simulink model "nonlineardtm"  (R2018b)
settings: configuration reference "Physics" (kept outside this file)
model workspace (MAT data in the model file):
  MCOS : class17 (value not decoded)
undefined symbols (not defined in the file): Aerodynamics, Aligning, Antisway, Brakes, Compliance, ContactPatch, Environment, k1_TireFB_PT1, k1_WheelsFB_PT1, k2_TireFB_PT1, Kinematics, Lateral, Longitudinal, normalizeAngle, omega0_K_Vehicle_radps, omega0_Wheels_radps, Overturning, p_Tires_Pa, Rolling, Scaling, SensorData, Structural, TireSimulation, Turnslip, v0_K_Vehicle_mps, v0z_Wheels_mps, VehicleData, Vertical, Wheels, x0_verticaldynamics, z0_TireDeflection_m
libraries: vehdynlibtire x4, vehdynlibsuspension x2, vrlib x1, vehdynlibeom x1
(part 3 of 5)

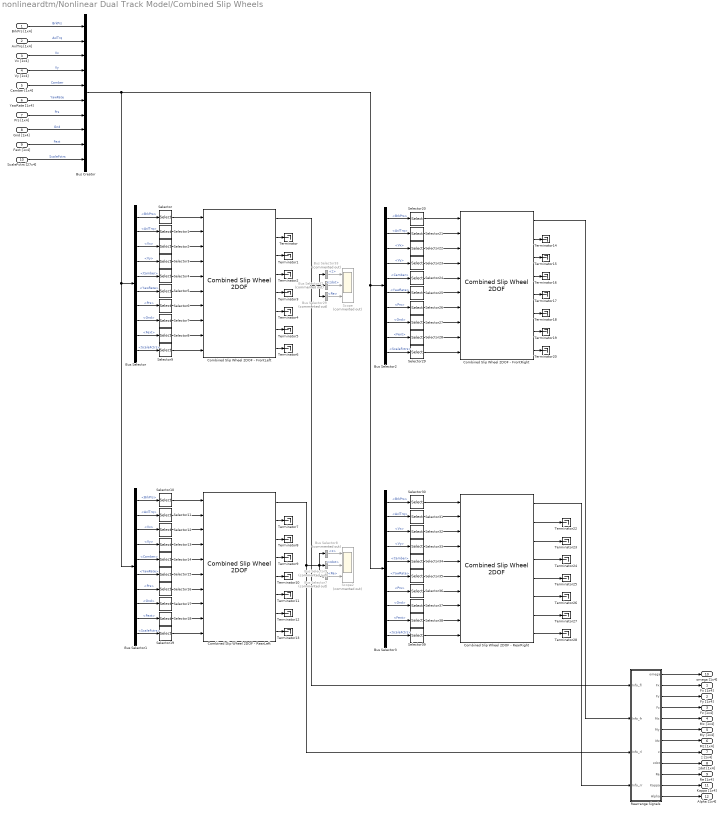
== system nonlineardtm/Nonlinear Dual Track Model/Combined Slip Wheels ==
  BrkPrs [1x4] : Inport
  AxlTrq [1x4] : Inport  Port=2
  Vx [1x4] : Inport  Port=3
  Vy [1x4] : Inport  Port=4
  Camber [1x4] : Inport  Port=5
  YawRate [1x4] : Inport  Port=6
  Prs [1x4] : Inport  Port=7
  Gnd [1x4] : Inport  Port=8
  Fext [1x4] : Inport  Port=9
  ScaleFctrs [27x4] : Inport  Port=10
  Bus Creator : BusCreator  Inputs=10
  Bus Selector{,1..3} (4 alike) : BusSelector  OutputSignals=BrkPrs,AxlTrq,Vx,Vy,Camber,YawRate,Prs,Gnd,Fext,ScaleFctrs
  Bus Selector29 : BusSelector  Commented=on  OutputSignals=Re
  Bus Selector33 : BusSelector  Commented=on  OutputSignals=z
  Bus Selector37 : BusSelector  Commented=on  OutputSignals=zdot
  Bus Selector7 : BusSelector  Commented=on  OutputSignals=Re
  Bus Selector8 : BusSelector  Commented=on  OutputSignals=z
  Bus Selector9 : BusSelector  Commented=on  OutputSignals=zdot
  Combined Slip Wheel 2DOF - FrontLeft : vehdynlibtire/Combined Slip Wheel 2DOF  BrakeType=Disc  mu_static=Brakes.mue_BrakePadsStaticFB (1)  mu_kinetic=Brakes.mue_BrakePadsKineticFB (1)  disk_abore=Brakes.d_BrakeBoreDiameterFB_m (1)  Rm=Brakes.r_BrakePadsMeanLeverRadiusFB_m (1)  num_pads=Brakes.n_BrakePadsNumberFB (1)  drum_abore=0.0508  drum_a=0.123  drum_c=0.212  drum_r=0.15  drum_theta1=0  drum_theta2=126  brake_p_bpt=[1 11.4736842105263 21.9473684210526 32.4210526315789 42.8947368421053 53.3684210526316 63.8421052631579 74.3157894736842 84.7894736842105 95.2631578947368 105.736842105263 116.210526315789 126.684210526316 137.157894736842 147.631578947368 158.105263157895 168.578947368421 179.052631578947 189.526315789474 200]  brake_n_bpt=[0 52.6315789473684 105.263157894737 157.894736842105 210.526315789474 263.157894736842 315.789473684211 368.421052631579 421.052631578947 473.684210526316 526.315789473684 578.947368421053 631.578947368421 684.210526315789 736.842105263158 789.473684210526 842.105263157895 894.736842105263 947.368421052632 1000]  f_brake_t=[43.4900602404453 42.5056030554862 41.5350898940194 40.5780454442085 39.6340111501808 38.7025443887544 37.7832176914519 36.8756180088306 35.9793460143796 35.0940154454303 34.2192524787115 33.3546951383474 32.4999927342521 31.6548053290159 30.8188032315107 29.991666515561 29.1730845621415 28.362755623661 27.5603864089927 26.765691687993;498.991217495636 487.695866636631 476.560505099801 465.579679307235 454.748127933653 444.060772460445 433.51270824929 423.099196101319 412.81565427025 402.657650900201 392.620896861006 382.701238955775 372.894653477208 363.197240090814 353.605216024701 344.114910546964 334.722759712992 325.425301366216 316.219170376863 307.10109410434;954.492374750826 932.886130217776 911.585920305583 890.581313170261 869.862244717126 849.419000532136 829.242198807128 809.322774193808 789.651962526121 770.221286354971 751.0225412433 732.047782773203 713.289314220164 694.739674852612 676.391628817892 658.238154578366 640.272434863842 622.48784710877 604.877954344734 587.436496520688;1409.99353200602 1378.07639379892 1346.61133551136 1315.58294703329 1284.9763615006 1254.77722860383 1224.97168936497 1195.5463522863 1166.48827078199 1137.78492180974 1109.42418562559 1081.39432659063 1053.68397496312 1026.28210961441 999.178041611083 972.361398609768 945.822110014692 919.550392851325 893.536738312604 867.771898937035;1865.49468926121 1823.26665738007 1781.63675071715 1740.58458089631 1700.09047828407 1660.13545667552 1620.7011799228 1581.76993037878 1543.32457903786 1505.34855726451 1467.82583000789 1430.74087040806 1394.07863570608 1357.82454437621 1321.96445440427 1286.48464264117 1251.37178516554 1216.61293859388 1182.19552228048 1148.10730135338;2320.9958465164 2268.45692096121 2216.66216592293 2165.58621475934 2115.20459506754 2065.49368474721 2016.43067048064 1967.99350847127 1920.16088729373 1872.91219271928 1826.22747439018 1780.08741422549 1734.47329644903 1689.36697913801 1644.75086719747 1600.60788667257 1556.92146031639 1513.67548433643 1470.85430624835 1428.44270376973;2776.49700377159 2713.64718454235 2651.68758112871 2590.58784862237 2530.31871185102 2470.8519128189 2412.16016103848 2354.21708656376 2296.9971955496 2240.47582817405 2184.62911877248 2129.43395804292 2074.86795719199 2020.9094138998 1967.53727999066 1914.73113070398 1862.47113546724 1810.73803007899 1759.51309021622 1708.77810618608;3231.99816102678 3158.8374481235 3086.71299633449 3015.58948248539 2945.43282863449 2876.21014089059 2807.88965159632 2740.44066465625 2673.83350380547 2608.03946362882 2543.03076315477 2478.78050186034 2415.26261793494 2352.4518486616 2290.32369278385 2228.85437473538 2168.02081061809 2107.80057582154 2048.17187418409 1989.11350860242;3687.49931828197 3604.02771170464 3521.73841154027 3440.59111634842 3360.54694541796 3281.56836896228 3203.61914215416 3126.66424274874 3050.66981206134 2975.60309908359 2901.43240753707 2828.12704567777 2755.6572786779 2683.9942834234 2613.11010557704 2542.97761876678 2473.57048576894 2404.8631215641 2336.83065815196 2269.44891101877;4143.00047553716 4049.21797528579 3956.76382674606 3865.59275021144 3775.66106220143 3686.92659703397 3599.34863271199 3512.88782084123 3427.50612031721 3343.16673453836 3259.83405191936 3177.4735894952 3096.05193942085 3015.5367181852 2935.89651837023 2857.10086279818 2779.12016091979 2701.92566730665 2625.48944211983 2549.78431343512;4598.50163279235 4494.40823886693 4391.78924195184 4290.59438407447 4190.77517898491 4092.28482510566 3995.07812326983 3899.11139893372 3804.34242857308 3710.73036999313 3618.23569630166 3526.82013331263 3436.44660016381 3347.079152947 3258.68293116342 3171.22410682959 3084.66983607064 2998.98821304921 2914.1482260877 2830.11971585147;5054.00279004754 4939.59850244808 4826.81465715762 4715.59601793749 4605.88929576838 4497.64305317735 4390.80761382767 4285.3349770262 4181.17873682896 4078.2940054479 3976.63734068395 3876.16667713006 3776.84126090677 3678.62158770879 3581.46934395661 3485.34735086099 ...(+2764 chars)]  tireParamSet=vdynPassCar.mat  plySteer=off  turnslip=off  PRESMAX=TireSimulation.PRESMAX(1)  PRESMIN=TireSimulation.PRESMIN(1)  FZMAX=TireSimulation.FZMAX(1)  FZMIN=TireSimulation.FZMIN(1)  VXLOW=TireSimulation.VXLOW(1)  KPUMAX=TireSimulation.KPUMAX(1)  KPUMIN=TireSimulation.KPUMIN(1)  ALPMAX=TireSimulation.ALPMAX(1)  ALPMIN=TireSimulation.ALPMIN(1)  CAMMAX=TireSimulation.CAMMAX(1)  CAMMIN=TireSimulation.CAMMIN(1)  LONGVL=TireSimulation.LONGVL(1)  omegao=omega0_Wheels_radps(1)  br=Wheels.mue_Wheels(1)  UNLOADED_RADIUS=Wheels.UNLOADED_RADIUS(1)  NOMPRES=Wheels.NOMPRES(1)  FNOMIN=Wheels.FNOMIN(1)  WIDTH=Wheels.WIDTH(1)  MASS=Wheels.m_WheelsFB_kg (1)  IYY=Wheels.Iyy_WheelsFB_kgm2 (1)  GRAVITY=- Wheels.a_Gravity_mps2  zo=z0_TireDeflection_m(1)  zdoto=v0z_Wheels_mps(1)  BREFF=Vertical.BREFF(1)  DREFF=Vertical.DREFF(1)  FREFF=Vertical.FREFF(1)  Q_RE0=Vertical.Q_RE0(1)  Q_V1=Vertical.Q_V1(1)  Q_V2=Vertical.Q_V2(1)  Q_FZ1=Vertical.Q_FZ1(1)  Q_FZ2=Vertical.Q_FZ2(1)  Q_FZ3=Vertical.Q_FZ3(1)  Q_FCX=Vertical.Q_FCX(1)  Q_FCY=Vertical.Q_FCY(1)  Q_FCY2=Vertical.Q_FCY2(1)  PFZ1=Vertical.PFZ1(1)  VERTICAL_STIFFNESS=Vertical.VERTICAL_STIFFNESS(1)  VERTICAL_DAMPING=Vertical.VERTICAL_DAMPING(1)  LONGITUDINAL_STIFFNESS=Structural.LONGITUDINAL_STIFFNESS(1)  LATERAL_STIFFNESS=Structural.LATERAL_STIFFNESS(1)  PCFX1=Structural.PCFX1(1)  PCFX2=Structural.PCFX2(1)  PCFX3=Structural.PCFX3(1)  PCFY1=Structural.PCFY1(1)  PCFY2=Structural.PCFY2(1)  PCFY3=Structural.PCFY3(1)  Q_RA1=ContactPatch.Q_RA1(1)  Q_RA2=ContactPatch.Q_RA2(1)  Q_RB1=ContactPatch.Q_RB1(1)  Q_RB2=ContactPatch.Q_RB2(1)  PCX1=Longitudinal.PCX1(1)  PDX1=Longitudinal.PDX1(1)  PDX2=Longitudinal.PDX2(1)  PDX3=Longitudinal.PDX3(1)  PEX1=Longitudinal.PEX1(1)  PEX2=Longitudinal.PEX2(1)  PEX3=Longitudinal.PEX3(1)  PEX4=Longitudinal.PEX4(1)  PKX1=Longitudinal.PKX1(1)  PKX2=Longitudinal.PKX2(1)  PKX3=Longitudinal.PKX3(1)  PHX1=Longitudinal.PHX1(1)  PHX2=Longitudinal.PHX2(1)  PVX1=Longitudinal.PVX1(1)  PVX2=Longitudinal.PVX2(1)  PPX1=Longitudinal.PPX1(1)  PPX2=Longitudinal.PPX2(1)  PPX3=Longitudinal.PPX3(1)  PPX4=Longitudinal.PPX4(1)  RBX1=Longitudinal.RBX1(1)  RBX2=Longitudinal.RBX2(1)  RBX3=Longitudinal.RBX3(1)  RCX1=Longitudinal.RCX1(1)  REX1=Longitudinal.REX1(1)  REX2=Longitudinal.REX2(1)  RHX1=Longitudinal.RHX1(1)  QSX1=Overturning.QSX1(1)  QSX2=Overturning.QSX2(1)  QSX3=Overturning.QSX3(1)  QSX4=Overturning.QSX4(1)  QSX5=Overturning.QSX5(1)  QSX6=Overturning.QSX6(1)  QSX7=Overturning.QSX7(1)  QSX8=Overturning.QSX8(1)  QSX9=Overturning.QSX9(1)  QSX10=Overturning.QSX10(1)  QSX11=Overturning.QSX11(1)  QSX12=Overturning.QSX12(1)  QSX13=Overturning.QSX13(1)  QSX14=Overturning.QSX14(1)  PPMX1=Overturning.PPMX1(1)  PCY1=Lateral.PCY1(1)  PDY1=Lateral.PDY1(1)  PDY2=Lateral.PDY2(1)  PDY3=Lateral.PDY3(1)  PEY1=Lateral.PEY1(1)  PEY2=Lateral.PEY2(1)  PEY3=Lateral.PEY3(1)  PEY4=Lateral.PEY4(1)  PEY5=Lateral.PEY5(1)  PKY1=Lateral.PKY1(1)  PKY2=Lateral.PKY2(1)  PKY3=Lateral.PKY3(1)  PKY4=Lateral.PKY4(1)  PKY5=Lateral.PKY5(1)  PKY6=Lateral.PKY6(1)  PKY7=Lateral.PKY7(1)  PHY1=Lateral.PHY1(1)  PHY2=Lateral.PHY2(1)  PVY1=Lateral.PVY1(1)  PVY2=Lateral.PVY2(1)  PVY3=Lateral.PVY3(1)  PVY4=Lateral.PVY4(1)  PPY1=Lateral.PPY1(1)  PPY2=Lateral.PPY2(1)  PPY3=Lateral.PPY3(1)  PPY4=Lateral.PPY4(1)  PPY5=Lateral.PPY5(1)  RBY1=Lateral.RBY1(1)  RBY2=Lateral.RBY2(1)  RBY3=Lateral.RBY3(1)  RBY4=Lateral.RBY4(1)  RCY1=Lateral.RCY1(1)  REY1=Lateral.REY1(1)  REY2=Lateral.REY2(1)  RHY1=Lateral.RHY1(1)  RHY2=Lateral.RHY2(1)  RVY1=Lateral.RVY1(1)  RVY2=Lateral.RVY2(1)  RVY3=Lateral.RVY3(1)  RVY4=Lateral.RVY4(1)  RVY5=Lateral.RVY5(1)  RVY6=Lateral.RVY6(1)  QSY1=Rolling.QSY1(1)  QSY2=Rolling.QSY2(1)  QSY3=Rolling.QSY3(1)  QSY4=Rolling.QSY4(1)  QSY5=Rolling.QSY5(1)  QSY6=Rolling.QSY6(1)  QSY7=Rolling.QSY7(1)  QSY8=Rolling.QSY8(1)  QBZ1=Aligning.QBZ1(1)  QBZ2=Aligning.QBZ2(1)  QBZ3=Aligning.QBZ3(1)  QBZ4=Aligning.QBZ4(1)  QBZ5=Aligning.QBZ5(1)  QBZ6=Aligning.QBZ6(1)  QBZ9=Aligning.QBZ9(1)  QBZ10=Aligning.QBZ10(1)  QCZ1=Aligning.QCZ1(1)  QDZ1=Aligning.QDZ1(1)  QDZ2=Aligning.QDZ2(1)  QDZ3=Aligning.QDZ3(1)  QDZ4=Aligning.QDZ4(1)  QDZ6=Aligning.QDZ6(1)  QDZ7=Aligning.QDZ7(1)  QDZ8=Aligning.QDZ8(1)  QDZ9=Aligning.QDZ9(1)  QDZ10=Aligning.QDZ10(1)  QDZ11=Aligning.QDZ11(1)  QEZ1=Aligning.QEZ1(1)  QEZ2=Aligning.QEZ2(1)  QEZ3=Aligning.QEZ3(1)  QEZ4=Aligning.QEZ4(1)  QEZ5=Aligning.QEZ5(1)  QHZ1=Aligning.QHZ1(1)  QHZ2=Aligning.QHZ2(1)  QHZ3=Aligning.QHZ3(1)  QHZ4=Aligning.QHZ4(1)  PPZ1=Aligning.PPZ1(1)  PPZ2=Aligning.PPZ2(1)  SSZ1=Aligning.SSZ1(1)  SSZ2=Aligning.SSZ2(1)  SSZ3=Aligning.SSZ3(1)  SSZ4=Aligning.SSZ4(1)  PDXP1=Turnslip.PDXP1(1)  PDXP2=Turnslip.PDXP2(1)  PDXP3=Turnslip.PDXP3(1)  PKYP1=Turnslip.PKYP1(1)  PDYP1=Turnslip.PDYP1(1)  PDYP2=Turnslip.PDYP2(1)  PDYP3=Turnslip.PDYP3(1)  PDYP4=Turnslip.PDYP4(1)  PHYP1=Turnslip.PHYP1(1)  PHYP2=Turnslip.PHYP2(1)  PHYP3=Turnslip.PHYP3(1)  PHYP4=Turnslip.PHYP4(1)  PECP1=Turnslip.PECP1(1)  PECP2=Turnslip.PECP2(1)  QDTP1=Turnslip.QDTP1(1)  QCRP1=Turnslip.QCRP1(1)  QCRP2=Turnslip.QCRP2(1)  QBRP1=Turnslip.QBRP1(1)  QDRP1=Turnslip.QDRP1(1)  QDRP2=Turnslip.QDRP2(1)  aMode=2
      settings: SourceProductName=Vehicle Dynamics Blockset  SourceProductBaseCode=VE
  Combined Slip Wheel 2DOF - FrontRight : vehdynlibtire/Combined Slip Wheel 2DOF  BrakeType=Disc  mu_static=Brakes.mue_BrakePadsStaticFB (1)  mu_kinetic=Brakes.mue_BrakePadsKineticFB (1)  disk_abore=Brakes.d_BrakeBoreDiameterFB_m (1)  Rm=Brakes.r_BrakePadsMeanLeverRadiusFB_m (1)  num_pads=Brakes.n_BrakePadsNumberFB (1)  drum_abore=0.0508  drum_a=0.123  drum_c=0.212  drum_r=0.15  drum_theta1=0  drum_theta2=126  brake_p_bpt=[1 11.4736842105263 21.9473684210526 32.4210526315789 42.8947368421053 53.3684210526316 63.8421052631579 74.3157894736842 84.7894736842105 95.2631578947368 105.736842105263 116.210526315789 126.684210526316 137.157894736842 147.631578947368 158.105263157895 168.578947368421 179.052631578947 189.526315789474 200]  brake_n_bpt=[0 52.6315789473684 105.263157894737 157.894736842105 210.526315789474 263.157894736842 315.789473684211 368.421052631579 421.052631578947 473.684210526316 526.315789473684 578.947368421053 631.578947368421 684.210526315789 736.842105263158 789.473684210526 842.105263157895 894.736842105263 947.368421052632 1000]  f_brake_t=[43.4900602404453 42.5056030554862 41.5350898940194 40.5780454442085 39.6340111501808 38.7025443887544 37.7832176914519 36.8756180088306 35.9793460143796 35.0940154454303 34.2192524787115 33.3546951383474 32.4999927342521 31.6548053290159 30.8188032315107 29.991666515561 29.1730845621415 28.362755623661 27.5603864089927 26.765691687993;498.991217495636 487.695866636631 476.560505099801 465.579679307235 454.748127933653 444.060772460445 433.51270824929 423.099196101319 412.81565427025 402.657650900201 392.620896861006 382.701238955775 372.894653477208 363.197240090814 353.605216024701 344.114910546964 334.722759712992 325.425301366216 316.219170376863 307.10109410434;954.492374750826 932.886130217776 911.585920305583 890.581313170261 869.862244717126 849.419000532136 829.242198807128 809.322774193808 789.651962526121 770.221286354971 751.0225412433 732.047782773203 713.289314220164 694.739674852612 676.391628817892 658.238154578366 640.272434863842 622.48784710877 604.877954344734 587.436496520688;1409.99353200602 1378.07639379892 1346.61133551136 1315.58294703329 1284.9763615006 1254.77722860383 1224.97168936497 1195.5463522863 1166.48827078199 1137.78492180974 1109.42418562559 1081.39432659063 1053.68397496312 1026.28210961441 999.178041611083 972.361398609768 945.822110014692 919.550392851325 893.536738312604 867.771898937035;1865.49468926121 1823.26665738007 1781.63675071715 1740.58458089631 1700.09047828407 1660.13545667552 1620.7011799228 1581.76993037878 1543.32457903786 1505.34855726451 1467.82583000789 1430.74087040806 1394.07863570608 1357.82454437621 1321.96445440427 1286.48464264117 1251.37178516554 1216.61293859388 1182.19552228048 1148.10730135338;2320.9958465164 2268.45692096121 2216.66216592293 2165.58621475934 2115.20459506754 2065.49368474721 2016.43067048064 1967.99350847127 1920.16088729373 1872.91219271928 1826.22747439018 1780.08741422549 1734.47329644903 1689.36697913801 1644.75086719747 1600.60788667257 1556.92146031639 1513.67548433643 1470.85430624835 1428.44270376973;2776.49700377159 2713.64718454235 2651.68758112871 2590.58784862237 2530.31871185102 2470.8519128189 2412.16016103848 2354.21708656376 2296.9971955496 2240.47582817405 2184.62911877248 2129.43395804292 2074.86795719199 2020.9094138998 1967.53727999066 1914.73113070398 1862.47113546724 1810.73803007899 1759.51309021622 1708.77810618608;3231.99816102678 3158.8374481235 3086.71299633449 3015.58948248539 2945.43282863449 2876.21014089059 2807.88965159632 2740.44066465625 2673.83350380547 2608.03946362882 2543.03076315477 2478.78050186034 2415.26261793494 2352.4518486616 2290.32369278385 2228.85437473538 2168.02081061809 2107.80057582154 2048.17187418409 1989.11350860242;3687.49931828197 3604.02771170464 3521.73841154027 3440.59111634842 3360.54694541796 3281.56836896228 3203.61914215416 3126.66424274874 3050.66981206134 2975.60309908359 2901.43240753707 2828.12704567777 2755.6572786779 2683.9942834234 2613.11010557704 2542.97761876678 2473.57048576894 2404.8631215641 2336.83065815196 2269.44891101877;4143.00047553716 4049.21797528579 3956.76382674606 3865.59275021144 3775.66106220143 3686.92659703397 3599.34863271199 3512.88782084123 3427.50612031721 3343.16673453836 3259.83405191936 3177.4735894952 3096.05193942085 3015.5367181852 2935.89651837023 2857.10086279818 2779.12016091979 2701.92566730665 2625.48944211983 2549.78431343512;4598.50163279235 4494.40823886693 4391.78924195184 4290.59438407447 4190.77517898491 4092.28482510566 3995.07812326983 3899.11139893372 3804.34242857308 3710.73036999313 3618.23569630166 3526.82013331263 3436.44660016381 3347.079152947 3258.68293116342 3171.22410682959 3084.66983607064 2998.98821304921 2914.1482260877 2830.11971585147;5054.00279004754 4939.59850244808 4826.81465715762 4715.59601793749 4605.88929576838 4497.64305317735 4390.80761382767 4285.3349770262 4181.17873682896 4078.2940054479 3976.63734068395 3876.16667713006 3776.84126090677 3678.62158770879 3581.46934395661 3485.34735086099 ...(+2764 chars)]  tireParamSet=vdynPassCar.mat  plySteer=off  turnslip=off  PRESMAX=TireSimulation.PRESMAX(2)  PRESMIN=TireSimulation.PRESMIN(2)  FZMAX=TireSimulation.FZMAX(2)  FZMIN=TireSimulation.FZMIN(2)  VXLOW=TireSimulation.VXLOW(2)  KPUMAX=TireSimulation.KPUMAX(2)  KPUMIN=TireSimulation.KPUMIN(2)  ALPMAX=TireSimulation.ALPMAX(2)  ALPMIN=TireSimulation.ALPMIN(2)  CAMMAX=TireSimulation.CAMMAX(2)  CAMMIN=TireSimulation.CAMMIN(2)  LONGVL=TireSimulation.LONGVL(2)  omegao=omega0_Wheels_radps(2)  br=Wheels.mue_Wheels(2)  UNLOADED_RADIUS=Wheels.UNLOADED_RADIUS(2)  NOMPRES=Wheels.NOMPRES(2)  FNOMIN=Wheels.FNOMIN(2)  WIDTH=Wheels.WIDTH(2)  MASS=Wheels.m_WheelsFB_kg (1)  IYY=Wheels.Iyy_WheelsFB_kgm2 (1)  GRAVITY=- Wheels.a_Gravity_mps2  zo=z0_TireDeflection_m(2)  zdoto=v0z_Wheels_mps(2)  BREFF=Vertical.BREFF(2)  DREFF=Vertical.DREFF(2)  FREFF=Vertical.FREFF(2)  Q_RE0=Vertical.Q_RE0(2)  Q_V1=Vertical.Q_V1(2)  Q_V2=Vertical.Q_V2(2)  Q_FZ1=Vertical.Q_FZ1(2)  Q_FZ2=Vertical.Q_FZ2(2)  Q_FZ3=Vertical.Q_FZ3(2)  Q_FCX=Vertical.Q_FCX(2)  Q_FCY=Vertical.Q_FCY(2)  Q_FCY2=Vertical.Q_FCY2(2)  PFZ1=Vertical.PFZ1(2)  VERTICAL_STIFFNESS=Vertical.VERTICAL_STIFFNESS(2)  VERTICAL_DAMPING=Vertical.VERTICAL_DAMPING(2)  LONGITUDINAL_STIFFNESS=Structural.LONGITUDINAL_STIFFNESS(2)  LATERAL_STIFFNESS=Structural.LATERAL_STIFFNESS(2)  PCFX1=Structural.PCFX1(2)  PCFX2=Structural.PCFX2(2)  PCFX3=Structural.PCFX3(2)  PCFY1=Structural.PCFY1(2)  PCFY2=Structural.PCFY2(2)  PCFY3=Structural.PCFY3(2)  Q_RA1=ContactPatch.Q_RA1(2)  Q_RA2=ContactPatch.Q_RA2(2)  Q_RB1=ContactPatch.Q_RB1(2)  Q_RB2=ContactPatch.Q_RB2(2)  PCX1=Longitudinal.PCX1(2)  PDX1=Longitudinal.PDX1(2)  PDX2=Longitudinal.PDX2(2)  PDX3=Longitudinal.PDX3(2)  PEX1=Longitudinal.PEX1(2)  PEX2=Longitudinal.PEX2(2)  PEX3=Longitudinal.PEX3(2)  PEX4=Longitudinal.PEX4(2)  PKX1=Longitudinal.PKX1(2)  PKX2=Longitudinal.PKX2(2)  PKX3=Longitudinal.PKX3(2)  PHX1=Longitudinal.PHX1(2)  PHX2=Longitudinal.PHX2(2)  PVX1=Longitudinal.PVX1(2)  PVX2=Longitudinal.PVX2(2)  PPX1=Longitudinal.PPX1(2)  PPX2=Longitudinal.PPX2(2)  PPX3=Longitudinal.PPX3(2)  PPX4=Longitudinal.PPX4(2)  RBX1=Longitudinal.RBX1(2)  RBX2=Longitudinal.RBX2(2)  RBX3=Longitudinal.RBX3(2)  RCX1=Longitudinal.RCX1(2)  REX1=Longitudinal.REX1(2)  REX2=Longitudinal.REX2(2)  RHX1=Longitudinal.RHX1(2)  QSX1=Overturning.QSX1(2)  QSX2=Overturning.QSX2(2)  QSX3=Overturning.QSX3(2)  QSX4=Overturning.QSX4(2)  QSX5=Overturning.QSX5(2)  QSX6=Overturning.QSX6(2)  QSX7=Overturning.QSX7(2)  QSX8=Overturning.QSX8(2)  QSX9=Overturning.QSX9(2)  QSX10=Overturning.QSX10(2)  QSX11=Overturning.QSX11(2)  QSX12=Overturning.QSX12(2)  QSX13=Overturning.QSX13(2)  QSX14=Overturning.QSX14(2)  PPMX1=Overturning.PPMX1(2)  PCY1=Lateral.PCY1(2)  PDY1=Lateral.PDY1(2)  PDY2=Lateral.PDY2(2)  PDY3=Lateral.PDY3(2)  PEY1=Lateral.PEY1(2)  PEY2=Lateral.PEY2(2)  PEY3=Lateral.PEY3(2)  PEY4=Lateral.PEY4(2)  PEY5=Lateral.PEY5(2)  PKY1=Lateral.PKY1(2)  PKY2=Lateral.PKY2(2)  PKY3=Lateral.PKY3(2)  PKY4=Lateral.PKY4(2)  PKY5=Lateral.PKY5(2)  PKY6=Lateral.PKY6(2)  PKY7=Lateral.PKY7(2)  PHY1=Lateral.PHY1(2)  PHY2=Lateral.PHY2(2)  PVY1=Lateral.PVY1(2)  PVY2=Lateral.PVY2(2)  PVY3=Lateral.PVY3(2)  PVY4=Lateral.PVY4(2)  PPY1=Lateral.PPY1(2)  PPY2=Lateral.PPY2(2)  PPY3=Lateral.PPY3(2)  PPY4=Lateral.PPY4(2)  PPY5=Lateral.PPY5(2)  RBY1=Lateral.RBY1(2)  RBY2=Lateral.RBY2(2)  RBY3=Lateral.RBY3(2)  RBY4=Lateral.RBY4(2)  RCY1=Lateral.RCY1(2)  REY1=Lateral.REY1(2)  REY2=Lateral.REY2(2)  RHY1=Lateral.RHY1(2)  RHY2=Lateral.RHY2(2)  RVY1=Lateral.RVY1(2)  RVY2=Lateral.RVY2(2)  RVY3=Lateral.RVY3(2)  RVY4=Lateral.RVY4(2)  RVY5=Lateral.RVY5(2)  RVY6=Lateral.RVY6(2)  QSY1=Rolling.QSY1(2)  QSY2=Rolling.QSY2(2)  QSY3=Rolling.QSY3(2)  QSY4=Rolling.QSY4(2)  QSY5=Rolling.QSY5(2)  QSY6=Rolling.QSY6(2)  QSY7=Rolling.QSY7(2)  QSY8=Rolling.QSY8(2)  QBZ1=Aligning.QBZ1(2)  QBZ2=Aligning.QBZ2(2)  QBZ3=Aligning.QBZ3(2)  QBZ4=Aligning.QBZ4(2)  QBZ5=Aligning.QBZ5(2)  QBZ6=Aligning.QBZ6(2)  QBZ9=Aligning.QBZ9(2)  QBZ10=Aligning.QBZ10(2)  QCZ1=Aligning.QCZ1(2)  QDZ1=Aligning.QDZ1(2)  QDZ2=Aligning.QDZ2(2)  QDZ3=Aligning.QDZ3(2)  QDZ4=Aligning.QDZ4(2)  QDZ6=Aligning.QDZ6(2)  QDZ7=Aligning.QDZ7(2)  QDZ8=Aligning.QDZ8(2)  QDZ9=Aligning.QDZ9(2)  QDZ10=Aligning.QDZ10(2)  QDZ11=Aligning.QDZ11(2)  QEZ1=Aligning.QEZ1(2)  QEZ2=Aligning.QEZ2(2)  QEZ3=Aligning.QEZ3(2)  QEZ4=Aligning.QEZ4(2)  QEZ5=Aligning.QEZ5(2)  QHZ1=Aligning.QHZ1(2)  QHZ2=Aligning.QHZ2(2)  QHZ3=Aligning.QHZ3(2)  QHZ4=Aligning.QHZ4(2)  PPZ1=Aligning.PPZ1(2)  PPZ2=Aligning.PPZ2(2)  SSZ1=Aligning.SSZ1(2)  SSZ2=Aligning.SSZ2(2)  SSZ3=Aligning.SSZ3(2)  SSZ4=Aligning.SSZ4(2)  PDXP1=Turnslip.PDXP1(2)  PDXP2=Turnslip.PDXP2(2)  PDXP3=Turnslip.PDXP3(2)  PKYP1=Turnslip.PKYP1(2)  PDYP1=Turnslip.PDYP1(2)  PDYP2=Turnslip.PDYP2(2)  PDYP3=Turnslip.PDYP3(2)  PDYP4=Turnslip.PDYP4(2)  PHYP1=Turnslip.PHYP1(2)  PHYP2=Turnslip.PHYP2(2)  PHYP3=Turnslip.PHYP3(2)  PHYP4=Turnslip.PHYP4(2)  PECP1=Turnslip.PECP1(2)  PECP2=Turnslip.PECP2(2)  QDTP1=Turnslip.QDTP1(2)  QCRP1=Turnslip.QCRP1(2)  QCRP2=Turnslip.QCRP2(2)  QBRP1=Turnslip.QBRP1(2)  QDRP1=Turnslip.QDRP1(2)  QDRP2=Turnslip.QDRP2(2)  aMode=2
      settings: SourceProductName=Vehicle Dynamics Blockset  SourceProductBaseCode=VE
  Combined Slip Wheel 2DOF - RearLeft : vehdynlibtire/Combined Slip Wheel 2DOF  BrakeType=Disc  mu_static=Brakes.mue_BrakePadsStaticFB (2)  mu_kinetic=Brakes.mue_BrakePadsKineticFB (2)  disk_abore=Brakes.d_BrakeBoreDiameterFB_m (2)  Rm=Brakes.r_BrakePadsMeanLeverRadiusFB_m (2)  num_pads=Brakes.n_BrakePadsNumberFB (2)  drum_abore=0.0508  drum_a=0.123  drum_c=0.212  drum_r=0.15  drum_theta1=0  drum_theta2=126  brake_p_bpt=[1 11.4736842105263 21.9473684210526 32.4210526315789 42.8947368421053 53.3684210526316 63.8421052631579 74.3157894736842 84.7894736842105 95.2631578947368 105.736842105263 116.210526315789 126.684210526316 137.157894736842 147.631578947368 158.105263157895 168.578947368421 179.052631578947 189.526315789474 200]  brake_n_bpt=[0 52.6315789473684 105.263157894737 157.894736842105 210.526315789474 263.157894736842 315.789473684211 368.421052631579 421.052631578947 473.684210526316 526.315789473684 578.947368421053 631.578947368421 684.210526315789 736.842105263158 789.473684210526 842.105263157895 894.736842105263 947.368421052632 1000]  f_brake_t=[43.4900602404453 42.5056030554862 41.5350898940194 40.5780454442085 39.6340111501808 38.7025443887544 37.7832176914519 36.8756180088306 35.9793460143796 35.0940154454303 34.2192524787115 33.3546951383474 32.4999927342521 31.6548053290159 30.8188032315107 29.991666515561 29.1730845621415 28.362755623661 27.5603864089927 26.765691687993;498.991217495636 487.695866636631 476.560505099801 465.579679307235 454.748127933653 444.060772460445 433.51270824929 423.099196101319 412.81565427025 402.657650900201 392.620896861006 382.701238955775 372.894653477208 363.197240090814 353.605216024701 344.114910546964 334.722759712992 325.425301366216 316.219170376863 307.10109410434;954.492374750826 932.886130217776 911.585920305583 890.581313170261 869.862244717126 849.419000532136 829.242198807128 809.322774193808 789.651962526121 770.221286354971 751.0225412433 732.047782773203 713.289314220164 694.739674852612 676.391628817892 658.238154578366 640.272434863842 622.48784710877 604.877954344734 587.436496520688;1409.99353200602 1378.07639379892 1346.61133551136 1315.58294703329 1284.9763615006 1254.77722860383 1224.97168936497 1195.5463522863 1166.48827078199 1137.78492180974 1109.42418562559 1081.39432659063 1053.68397496312 1026.28210961441 999.178041611083 972.361398609768 945.822110014692 919.550392851325 893.536738312604 867.771898937035;1865.49468926121 1823.26665738007 1781.63675071715 1740.58458089631 1700.09047828407 1660.13545667552 1620.7011799228 1581.76993037878 1543.32457903786 1505.34855726451 1467.82583000789 1430.74087040806 1394.07863570608 1357.82454437621 1321.96445440427 1286.48464264117 1251.37178516554 1216.61293859388 1182.19552228048 1148.10730135338;2320.9958465164 2268.45692096121 2216.66216592293 2165.58621475934 2115.20459506754 2065.49368474721 2016.43067048064 1967.99350847127 1920.16088729373 1872.91219271928 1826.22747439018 1780.08741422549 1734.47329644903 1689.36697913801 1644.75086719747 1600.60788667257 1556.92146031639 1513.67548433643 1470.85430624835 1428.44270376973;2776.49700377159 2713.64718454235 2651.68758112871 2590.58784862237 2530.31871185102 2470.8519128189 2412.16016103848 2354.21708656376 2296.9971955496 2240.47582817405 2184.62911877248 2129.43395804292 2074.86795719199 2020.9094138998 1967.53727999066 1914.73113070398 1862.47113546724 1810.73803007899 1759.51309021622 1708.77810618608;3231.99816102678 3158.8374481235 3086.71299633449 3015.58948248539 2945.43282863449 2876.21014089059 2807.88965159632 2740.44066465625 2673.83350380547 2608.03946362882 2543.03076315477 2478.78050186034 2415.26261793494 2352.4518486616 2290.32369278385 2228.85437473538 2168.02081061809 2107.80057582154 2048.17187418409 1989.11350860242;3687.49931828197 3604.02771170464 3521.73841154027 3440.59111634842 3360.54694541796 3281.56836896228 3203.61914215416 3126.66424274874 3050.66981206134 2975.60309908359 2901.43240753707 2828.12704567777 2755.6572786779 2683.9942834234 2613.11010557704 2542.97761876678 2473.57048576894 2404.8631215641 2336.83065815196 2269.44891101877;4143.00047553716 4049.21797528579 3956.76382674606 3865.59275021144 3775.66106220143 3686.92659703397 3599.34863271199 3512.88782084123 3427.50612031721 3343.16673453836 3259.83405191936 3177.4735894952 3096.05193942085 3015.5367181852 2935.89651837023 2857.10086279818 2779.12016091979 2701.92566730665 2625.48944211983 2549.78431343512;4598.50163279235 4494.40823886693 4391.78924195184 4290.59438407447 4190.77517898491 4092.28482510566 3995.07812326983 3899.11139893372 3804.34242857308 3710.73036999313 3618.23569630166 3526.82013331263 3436.44660016381 3347.079152947 3258.68293116342 3171.22410682959 3084.66983607064 2998.98821304921 2914.1482260877 2830.11971585147;5054.00279004754 4939.59850244808 4826.81465715762 4715.59601793749 4605.88929576838 4497.64305317735 4390.80761382767 4285.3349770262 4181.17873682896 4078.2940054479 3976.63734068395 3876.16667713006 3776.84126090677 3678.62158770879 3581.46934395661 3485.34735086099 ...(+2764 chars)]  tireParamSet=vdynPassCar.mat  plySteer=off  turnslip=off  PRESMAX=TireSimulation.PRESMAX(3)  PRESMIN=TireSimulation.PRESMIN(3)  FZMAX=TireSimulation.FZMAX(3)  FZMIN=TireSimulation.FZMIN(3)  VXLOW=TireSimulation.VXLOW(3)  KPUMAX=TireSimulation.KPUMAX(3)  KPUMIN=TireSimulation.KPUMIN(3)  ALPMAX=TireSimulation.ALPMAX(3)  ALPMIN=TireSimulation.ALPMIN(3)  CAMMAX=TireSimulation.CAMMAX(3)  CAMMIN=TireSimulation.CAMMIN(3)  LONGVL=TireSimulation.LONGVL(3)  omegao=omega0_Wheels_radps(3)  br=Wheels.mue_Wheels(3)  UNLOADED_RADIUS=Wheels.UNLOADED_RADIUS(3)  NOMPRES=Wheels.NOMPRES(3)  FNOMIN=Wheels.FNOMIN(3)  WIDTH=Wheels.WIDTH(3)  MASS=Wheels.m_WheelsFB_kg (2)  IYY=Wheels.Iyy_WheelsFB_kgm2 (2)  GRAVITY=- Wheels.a_Gravity_mps2  zo=z0_TireDeflection_m(3)  zdoto=v0z_Wheels_mps(3)  BREFF=Vertical.BREFF(3)  DREFF=Vertical.DREFF(3)  FREFF=Vertical.FREFF(3)  Q_RE0=Vertical.Q_RE0(3)  Q_V1=Vertical.Q_V1(3)  Q_V2=Vertical.Q_V2(3)  Q_FZ1=Vertical.Q_FZ1(3)  Q_FZ2=Vertical.Q_FZ2(3)  Q_FZ3=Vertical.Q_FZ3(3)  Q_FCX=Vertical.Q_FCX(3)  Q_FCY=Vertical.Q_FCY(3)  Q_FCY2=Vertical.Q_FCY2(3)  PFZ1=Vertical.PFZ1(3)  VERTICAL_STIFFNESS=Vertical.VERTICAL_STIFFNESS(3)  VERTICAL_DAMPING=Vertical.VERTICAL_DAMPING(3)  LONGITUDINAL_STIFFNESS=Structural.LONGITUDINAL_STIFFNESS(3)  LATERAL_STIFFNESS=Structural.LATERAL_STIFFNESS(3)  PCFX1=Structural.PCFX1(3)  PCFX2=Structural.PCFX2(3)  PCFX3=Structural.PCFX3(3)  PCFY1=Structural.PCFY1(3)  PCFY2=Structural.PCFY2(3)  PCFY3=Structural.PCFY3(3)  Q_RA1=ContactPatch.Q_RA1(3)  Q_RA2=ContactPatch.Q_RA2(3)  Q_RB1=ContactPatch.Q_RB1(3)  Q_RB2=ContactPatch.Q_RB2(3)  PCX1=Longitudinal.PCX1(3)  PDX1=Longitudinal.PDX1(3)  PDX2=Longitudinal.PDX2(3)  PDX3=Longitudinal.PDX3(3)  PEX1=Longitudinal.PEX1(3)  PEX2=Longitudinal.PEX2(3)  PEX3=Longitudinal.PEX3(3)  PEX4=Longitudinal.PEX4(3)  PKX1=Longitudinal.PKX1(3)  PKX2=Longitudinal.PKX2(3)  PKX3=Longitudinal.PKX3(3)  PHX1=Longitudinal.PHX1(3)  PHX2=Longitudinal.PHX2(3)  PVX1=Longitudinal.PVX1(3)  PVX2=Longitudinal.PVX2(3)  PPX1=Longitudinal.PPX1(3)  PPX2=Longitudinal.PPX2(3)  PPX3=Longitudinal.PPX3(3)  PPX4=Longitudinal.PPX4(3)  RBX1=Longitudinal.RBX1(3)  RBX2=Longitudinal.RBX2(3)  RBX3=Longitudinal.RBX3(3)  RCX1=Longitudinal.RCX1(3)  REX1=Longitudinal.REX1(3)  REX2=Longitudinal.REX2(3)  RHX1=Longitudinal.RHX1(3)  QSX1=Overturning.QSX1(3)  QSX2=Overturning.QSX2(3)  QSX3=Overturning.QSX3(3)  QSX4=Overturning.QSX4(3)  QSX5=Overturning.QSX5(3)  QSX6=Overturning.QSX6(3)  QSX7=Overturning.QSX7(3)  QSX8=Overturning.QSX8(3)  QSX9=Overturning.QSX9(3)  QSX10=Overturning.QSX10(3)  QSX11=Overturning.QSX11(3)  QSX12=Overturning.QSX12(3)  QSX13=Overturning.QSX13(3)  QSX14=Overturning.QSX14(3)  PPMX1=Overturning.PPMX1(3)  PCY1=Lateral.PCY1(3)  PDY1=Lateral.PDY1(3)  PDY2=Lateral.PDY2(3)  PDY3=Lateral.PDY3(3)  PEY1=Lateral.PEY1(3)  PEY2=Lateral.PEY2(3)  PEY3=Lateral.PEY3(3)  PEY4=Lateral.PEY4(3)  PEY5=Lateral.PEY5(3)  PKY1=Lateral.PKY1(3)  PKY2=Lateral.PKY2(3)  PKY3=Lateral.PKY3(3)  PKY4=Lateral.PKY4(3)  PKY5=Lateral.PKY5(3)  PKY6=Lateral.PKY6(3)  PKY7=Lateral.PKY7(3)  PHY1=Lateral.PHY1(3)  PHY2=Lateral.PHY2(3)  PVY1=Lateral.PVY1(3)  PVY2=Lateral.PVY2(3)  PVY3=Lateral.PVY3(3)  PVY4=Lateral.PVY4(3)  PPY1=Lateral.PPY1(3)  PPY2=Lateral.PPY2(3)  PPY3=Lateral.PPY3(3)  PPY4=Lateral.PPY4(3)  PPY5=Lateral.PPY5(3)  RBY1=Lateral.RBY1(3)  RBY2=Lateral.RBY2(3)  RBY3=Lateral.RBY3(3)  RBY4=Lateral.RBY4(3)  RCY1=Lateral.RCY1(3)  REY1=Lateral.REY1(3)  REY2=Lateral.REY2(3)  RHY1=Lateral.RHY1(3)  RHY2=Lateral.RHY2(3)  RVY1=Lateral.RVY1(3)  RVY2=Lateral.RVY2(3)  RVY3=Lateral.RVY3(3)  RVY4=Lateral.RVY4(3)  RVY5=Lateral.RVY5(3)  RVY6=Lateral.RVY6(3)  QSY1=Rolling.QSY1(3)  QSY2=Rolling.QSY2(3)  QSY3=Rolling.QSY3(3)  QSY4=Rolling.QSY4(3)  QSY5=Rolling.QSY5(3)  QSY6=Rolling.QSY6(3)  QSY7=Rolling.QSY7(3)  QSY8=Rolling.QSY8(3)  QBZ1=Aligning.QBZ1(3)  QBZ2=Aligning.QBZ2(3)  QBZ3=Aligning.QBZ3(3)  QBZ4=Aligning.QBZ4(3)  QBZ5=Aligning.QBZ5(3)  QBZ6=Aligning.QBZ6(3)  QBZ9=Aligning.QBZ9(3)  QBZ10=Aligning.QBZ10(3)  QCZ1=Aligning.QCZ1(3)  QDZ1=Aligning.QDZ1(3)  QDZ2=Aligning.QDZ2(3)  QDZ3=Aligning.QDZ3(3)  QDZ4=Aligning.QDZ4(3)  QDZ6=Aligning.QDZ6(3)  QDZ7=Aligning.QDZ7(3)  QDZ8=Aligning.QDZ8(3)  QDZ9=Aligning.QDZ9(3)  QDZ10=Aligning.QDZ10(3)  QDZ11=Aligning.QDZ11(3)  QEZ1=Aligning.QEZ1(3)  QEZ2=Aligning.QEZ2(3)  QEZ3=Aligning.QEZ3(3)  QEZ4=Aligning.QEZ4(3)  QEZ5=Aligning.QEZ5(3)  QHZ1=Aligning.QHZ1(3)  QHZ2=Aligning.QHZ2(3)  QHZ3=Aligning.QHZ3(3)  QHZ4=Aligning.QHZ4(3)  PPZ1=Aligning.PPZ1(3)  PPZ2=Aligning.PPZ2(3)  SSZ1=Aligning.SSZ1(3)  SSZ2=Aligning.SSZ2(3)  SSZ3=Aligning.SSZ3(3)  SSZ4=Aligning.SSZ4(3)  PDXP1=Turnslip.PDXP1(3)  PDXP2=Turnslip.PDXP2(3)  PDXP3=Turnslip.PDXP3(3)  PKYP1=Turnslip.PKYP1(3)  PDYP1=Turnslip.PDYP1(3)  PDYP2=Turnslip.PDYP2(3)  PDYP3=Turnslip.PDYP3(3)  PDYP4=Turnslip.PDYP4(3)  PHYP1=Turnslip.PHYP1(3)  PHYP2=Turnslip.PHYP2(3)  PHYP3=Turnslip.PHYP3(3)  PHYP4=Turnslip.PHYP4(3)  PECP1=Turnslip.PECP1(3)  PECP2=Turnslip.PECP2(3)  QDTP1=Turnslip.QDTP1(3)  QCRP1=Turnslip.QCRP1(3)  QCRP2=Turnslip.QCRP2(3)  QBRP1=Turnslip.QBRP1(3)  QDRP1=Turnslip.QDRP1(3)  QDRP2=Turnslip.QDRP2(3)  aMode=2
      settings: SourceProductName=Vehicle Dynamics Blockset  SourceProductBaseCode=VE
  Combined Slip Wheel 2DOF - RearRight : vehdynlibtire/Combined Slip Wheel 2DOF  BrakeType=Disc  mu_static=Brakes.mue_BrakePadsStaticFB (2)  mu_kinetic=Brakes.mue_BrakePadsKineticFB (2)  disk_abore=Brakes.d_BrakeBoreDiameterFB_m (2)  Rm=Brakes.r_BrakePadsMeanLeverRadiusFB_m (2)  num_pads=Brakes.n_BrakePadsNumberFB (2)  drum_abore=0.0508  drum_a=0.123  drum_c=0.212  drum_r=0.15  drum_theta1=0  drum_theta2=126  brake_p_bpt=[1 11.4736842105263 21.9473684210526 32.4210526315789 42.8947368421053 53.3684210526316 63.8421052631579 74.3157894736842 84.7894736842105 95.2631578947368 105.736842105263 116.210526315789 126.684210526316 137.157894736842 147.631578947368 158.105263157895 168.578947368421 179.052631578947 189.526315789474 200]  brake_n_bpt=[0 52.6315789473684 105.263157894737 157.894736842105 210.526315789474 263.157894736842 315.789473684211 368.421052631579 421.052631578947 473.684210526316 526.315789473684 578.947368421053 631.578947368421 684.210526315789 736.842105263158 789.473684210526 842.105263157895 894.736842105263 947.368421052632 1000]  f_brake_t=[43.4900602404453 42.5056030554862 41.5350898940194 40.5780454442085 39.6340111501808 38.7025443887544 37.7832176914519 36.8756180088306 35.9793460143796 35.0940154454303 34.2192524787115 33.3546951383474 32.4999927342521 31.6548053290159 30.8188032315107 29.991666515561 29.1730845621415 28.362755623661 27.5603864089927 26.765691687993;498.991217495636 487.695866636631 476.560505099801 465.579679307235 454.748127933653 444.060772460445 433.51270824929 423.099196101319 412.81565427025 402.657650900201 392.620896861006 382.701238955775 372.894653477208 363.197240090814 353.605216024701 344.114910546964 334.722759712992 325.425301366216 316.219170376863 307.10109410434;954.492374750826 932.886130217776 911.585920305583 890.581313170261 869.862244717126 849.419000532136 829.242198807128 809.322774193808 789.651962526121 770.221286354971 751.0225412433 732.047782773203 713.289314220164 694.739674852612 676.391628817892 658.238154578366 640.272434863842 622.48784710877 604.877954344734 587.436496520688;1409.99353200602 1378.07639379892 1346.61133551136 1315.58294703329 1284.9763615006 1254.77722860383 1224.97168936497 1195.5463522863 1166.48827078199 1137.78492180974 1109.42418562559 1081.39432659063 1053.68397496312 1026.28210961441 999.178041611083 972.361398609768 945.822110014692 919.550392851325 893.536738312604 867.771898937035;1865.49468926121 1823.26665738007 1781.63675071715 1740.58458089631 1700.09047828407 1660.13545667552 1620.7011799228 1581.76993037878 1543.32457903786 1505.34855726451 1467.82583000789 1430.74087040806 1394.07863570608 1357.82454437621 1321.96445440427 1286.48464264117 1251.37178516554 1216.61293859388 1182.19552228048 1148.10730135338;2320.9958465164 2268.45692096121 2216.66216592293 2165.58621475934 2115.20459506754 2065.49368474721 2016.43067048064 1967.99350847127 1920.16088729373 1872.91219271928 1826.22747439018 1780.08741422549 1734.47329644903 1689.36697913801 1644.75086719747 1600.60788667257 1556.92146031639 1513.67548433643 1470.85430624835 1428.44270376973;2776.49700377159 2713.64718454235 2651.68758112871 2590.58784862237 2530.31871185102 2470.8519128189 2412.16016103848 2354.21708656376 2296.9971955496 2240.47582817405 2184.62911877248 2129.43395804292 2074.86795719199 2020.9094138998 1967.53727999066 1914.73113070398 1862.47113546724 1810.73803007899 1759.51309021622 1708.77810618608;3231.99816102678 3158.8374481235 3086.71299633449 3015.58948248539 2945.43282863449 2876.21014089059 2807.88965159632 2740.44066465625 2673.83350380547 2608.03946362882 2543.03076315477 2478.78050186034 2415.26261793494 2352.4518486616 2290.32369278385 2228.85437473538 2168.02081061809 2107.80057582154 2048.17187418409 1989.11350860242;3687.49931828197 3604.02771170464 3521.73841154027 3440.59111634842 3360.54694541796 3281.56836896228 3203.61914215416 3126.66424274874 3050.66981206134 2975.60309908359 2901.43240753707 2828.12704567777 2755.6572786779 2683.9942834234 2613.11010557704 2542.97761876678 2473.57048576894 2404.8631215641 2336.83065815196 2269.44891101877;4143.00047553716 4049.21797528579 3956.76382674606 3865.59275021144 3775.66106220143 3686.92659703397 3599.34863271199 3512.88782084123 3427.50612031721 3343.16673453836 3259.83405191936 3177.4735894952 3096.05193942085 3015.5367181852 2935.89651837023 2857.10086279818 2779.12016091979 2701.92566730665 2625.48944211983 2549.78431343512;4598.50163279235 4494.40823886693 4391.78924195184 4290.59438407447 4190.77517898491 4092.28482510566 3995.07812326983 3899.11139893372 3804.34242857308 3710.73036999313 3618.23569630166 3526.82013331263 3436.44660016381 3347.079152947 3258.68293116342 3171.22410682959 3084.66983607064 2998.98821304921 2914.1482260877 2830.11971585147;5054.00279004754 4939.59850244808 4826.81465715762 4715.59601793749 4605.88929576838 4497.64305317735 4390.80761382767 4285.3349770262 4181.17873682896 4078.2940054479 3976.63734068395 3876.16667713006 3776.84126090677 3678.62158770879 3581.46934395661 3485.34735086099 ...(+2764 chars)]  tireParamSet=vdynPassCar.mat  plySteer=off  turnslip=off  PRESMAX=TireSimulation.PRESMAX(4)  PRESMIN=TireSimulation.PRESMIN(4)  FZMAX=TireSimulation.FZMAX(4)  FZMIN=TireSimulation.FZMIN(4)  VXLOW=TireSimulation.VXLOW(4)  KPUMAX=TireSimulation.KPUMAX(4)  KPUMIN=TireSimulation.KPUMIN(4)  ALPMAX=TireSimulation.ALPMAX(4)  ALPMIN=TireSimulation.ALPMIN(4)  CAMMAX=TireSimulation.CAMMAX(4)  CAMMIN=TireSimulation.CAMMIN(4)  LONGVL=TireSimulation.LONGVL(4)  omegao=omega0_Wheels_radps(4)  br=Wheels.mue_Wheels(4)  UNLOADED_RADIUS=Wheels.UNLOADED_RADIUS(4)  NOMPRES=Wheels.NOMPRES(4)  FNOMIN=Wheels.FNOMIN(4)  WIDTH=Wheels.WIDTH(4)  MASS=Wheels.m_WheelsFB_kg (2)  IYY=Wheels.Iyy_WheelsFB_kgm2 (2)  GRAVITY=- Wheels.a_Gravity_mps2  zo=z0_TireDeflection_m(4)  zdoto=v0z_Wheels_mps(4)  BREFF=Vertical.BREFF(4)  DREFF=Vertical.DREFF(4)  FREFF=Vertical.FREFF(4)  Q_RE0=Vertical.Q_RE0(4)  Q_V1=Vertical.Q_V1(4)  Q_V2=Vertical.Q_V2(4)  Q_FZ1=Vertical.Q_FZ1(4)  Q_FZ2=Vertical.Q_FZ2(4)  Q_FZ3=Vertical.Q_FZ3(4)  Q_FCX=Vertical.Q_FCX(4)  Q_FCY=Vertical.Q_FCY(4)  Q_FCY2=Vertical.Q_FCY2(4)  PFZ1=Vertical.PFZ1(4)  VERTICAL_STIFFNESS=Vertical.VERTICAL_STIFFNESS(4)  VERTICAL_DAMPING=Vertical.VERTICAL_DAMPING(4)  LONGITUDINAL_STIFFNESS=Structural.LONGITUDINAL_STIFFNESS(4)  LATERAL_STIFFNESS=Structural.LATERAL_STIFFNESS(4)  PCFX1=Structural.PCFX1(4)  PCFX2=Structural.PCFX2(4)  PCFX3=Structural.PCFX3(4)  PCFY1=Structural.PCFY1(4)  PCFY2=Structural.PCFY2(4)  PCFY3=Structural.PCFY3(4)  Q_RA1=ContactPatch.Q_RA1(4)  Q_RA2=ContactPatch.Q_RA2(4)  Q_RB1=ContactPatch.Q_RB1(4)  Q_RB2=ContactPatch.Q_RB2(4)  PCX1=Longitudinal.PCX1(4)  PDX1=Longitudinal.PDX1(4)  PDX2=Longitudinal.PDX2(4)  PDX3=Longitudinal.PDX3(4)  PEX1=Longitudinal.PEX1(4)  PEX2=Longitudinal.PEX2(4)  PEX3=Longitudinal.PEX3(4)  PEX4=Longitudinal.PEX4(4)  PKX1=Longitudinal.PKX1(4)  PKX2=Longitudinal.PKX2(4)  PKX3=Longitudinal.PKX3(4)  PHX1=Longitudinal.PHX1(4)  PHX2=Longitudinal.PHX2(4)  PVX1=Longitudinal.PVX1(4)  PVX2=Longitudinal.PVX2(4)  PPX1=Longitudinal.PPX1(4)  PPX2=Longitudinal.PPX2(4)  PPX3=Longitudinal.PPX3(4)  PPX4=Longitudinal.PPX4(4)  RBX1=Longitudinal.RBX1(4)  RBX2=Longitudinal.RBX2(4)  RBX3=Longitudinal.RBX3(4)  RCX1=Longitudinal.RCX1(4)  REX1=Longitudinal.REX1(4)  REX2=Longitudinal.REX2(4)  RHX1=Longitudinal.RHX1(4)  QSX1=Overturning.QSX1(4)  QSX2=Overturning.QSX2(4)  QSX3=Overturning.QSX3(4)  QSX4=Overturning.QSX4(4)  QSX5=Overturning.QSX5(4)  QSX6=Overturning.QSX6(4)  QSX7=Overturning.QSX7(4)  QSX8=Overturning.QSX8(4)  QSX9=Overturning.QSX9(4)  QSX10=Overturning.QSX10(4)  QSX11=Overturning.QSX11(4)  QSX12=Overturning.QSX12(4)  QSX13=Overturning.QSX13(4)  QSX14=Overturning.QSX14(4)  PPMX1=Overturning.PPMX1(4)  PCY1=Lateral.PCY1(4)  PDY1=Lateral.PDY1(4)  PDY2=Lateral.PDY2(4)  PDY3=Lateral.PDY3(4)  PEY1=Lateral.PEY1(4)  PEY2=Lateral.PEY2(4)  PEY3=Lateral.PEY3(4)  PEY4=Lateral.PEY4(4)  PEY5=Lateral.PEY5(4)  PKY1=Lateral.PKY1(4)  PKY2=Lateral.PKY2(4)  PKY3=Lateral.PKY3(4)  PKY4=Lateral.PKY4(4)  PKY5=Lateral.PKY5(4)  PKY6=Lateral.PKY6(4)  PKY7=Lateral.PKY7(4)  PHY1=Lateral.PHY1(4)  PHY2=Lateral.PHY2(4)  PVY1=Lateral.PVY1(4)  PVY2=Lateral.PVY2(4)  PVY3=Lateral.PVY3(4)  PVY4=Lateral.PVY4(4)  PPY1=Lateral.PPY1(4)  PPY2=Lateral.PPY2(4)  PPY3=Lateral.PPY3(4)  PPY4=Lateral.PPY4(4)  PPY5=Lateral.PPY5(4)  RBY1=Lateral.RBY1(4)  RBY2=Lateral.RBY2(4)  RBY3=Lateral.RBY3(4)  RBY4=Lateral.RBY4(4)  RCY1=Lateral.RCY1(4)  REY1=Lateral.REY1(4)  REY2=Lateral.REY2(4)  RHY1=Lateral.RHY1(4)  RHY2=Lateral.RHY2(4)  RVY1=Lateral.RVY1(4)  RVY2=Lateral.RVY2(4)  RVY3=Lateral.RVY3(4)  RVY4=Lateral.RVY4(4)  RVY5=Lateral.RVY5(4)  RVY6=Lateral.RVY6(4)  QSY1=Rolling.QSY1(4)  QSY2=Rolling.QSY2(4)  QSY3=Rolling.QSY3(4)  QSY4=Rolling.QSY4(4)  QSY5=Rolling.QSY5(4)  QSY6=Rolling.QSY6(4)  QSY7=Rolling.QSY7(4)  QSY8=Rolling.QSY8(4)  QBZ1=Aligning.QBZ1(4)  QBZ2=Aligning.QBZ2(4)  QBZ3=Aligning.QBZ3(4)  QBZ4=Aligning.QBZ4(4)  QBZ5=Aligning.QBZ5(4)  QBZ6=Aligning.QBZ6(4)  QBZ9=Aligning.QBZ9(4)  QBZ10=Aligning.QBZ10(4)  QCZ1=Aligning.QCZ1(4)  QDZ1=Aligning.QDZ1(4)  QDZ2=Aligning.QDZ2(4)  QDZ3=Aligning.QDZ3(4)  QDZ4=Aligning.QDZ4(4)  QDZ6=Aligning.QDZ6(4)  QDZ7=Aligning.QDZ7(4)  QDZ8=Aligning.QDZ8(4)  QDZ9=Aligning.QDZ9(4)  QDZ10=Aligning.QDZ10(4)  QDZ11=Aligning.QDZ11(4)  QEZ1=Aligning.QEZ1(4)  QEZ2=Aligning.QEZ2(4)  QEZ3=Aligning.QEZ3(4)  QEZ4=Aligning.QEZ4(4)  QEZ5=Aligning.QEZ5(4)  QHZ1=Aligning.QHZ1(4)  QHZ2=Aligning.QHZ2(4)  QHZ3=Aligning.QHZ3(4)  QHZ4=Aligning.QHZ4(4)  PPZ1=Aligning.PPZ1(4)  PPZ2=Aligning.PPZ2(4)  SSZ1=Aligning.SSZ1(4)  SSZ2=Aligning.SSZ2(4)  SSZ3=Aligning.SSZ3(4)  SSZ4=Aligning.SSZ4(4)  PDXP1=Turnslip.PDXP1(4)  PDXP2=Turnslip.PDXP2(4)  PDXP3=Turnslip.PDXP3(4)  PKYP1=Turnslip.PKYP1(4)  PDYP1=Turnslip.PDYP1(4)  PDYP2=Turnslip.PDYP2(4)  PDYP3=Turnslip.PDYP3(4)  PDYP4=Turnslip.PDYP4(4)  PHYP1=Turnslip.PHYP1(4)  PHYP2=Turnslip.PHYP2(4)  PHYP3=Turnslip.PHYP3(4)  PHYP4=Turnslip.PHYP4(4)  PECP1=Turnslip.PECP1(4)  PECP2=Turnslip.PECP2(4)  QDTP1=Turnslip.QDTP1(4)  QCRP1=Turnslip.QCRP1(4)  QCRP2=Turnslip.QCRP2(4)  QBRP1=Turnslip.QBRP1(4)  QDRP1=Turnslip.QDRP1(4)  QDRP2=Turnslip.QDRP2(4)  aMode=2
      settings: SourceProductName=Vehicle Dynamics Blockset  SourceProductBaseCode=VE
  Rearrange Signals : Subsystem
  Scope : Scope  Commented=on  NumInputPorts=3
  Scope2 : Scope  Commented=on  NumInputPorts=3
  Selector{,1..8} (9 alike) : Selector  InputPortWidth=4  IndexOptions=Index vector (dialog)  Indices=1  OutputSizes=1
  Selector{10..18} (9 alike) : Selector  InputPortWidth=4  IndexOptions=Index vector (dialog)  Indices=3  OutputSizes=1
  Selector19 : Selector  NumberOfDimensions=2  InputPortWidth=4  IndexOptions=Select all,Index vector (dialog)  Indices=3,3  OutputSizes=1,1
  Selector{20..28} (9 alike) : Selector  InputPortWidth=4  IndexOptions=Index vector (dialog)  Indices=2  OutputSizes=1
  Selector29 : Selector  NumberOfDimensions=2  InputPortWidth=4  IndexOptions=Select all,Index vector (dialog)  Indices=2,2  OutputSizes=1,1
  Selector{30..38} (9 alike) : Selector  InputPortWidth=4  IndexOptions=Index vector (dialog)  Indices=4  OutputSizes=1
  Selector39 : Selector  NumberOfDimensions=2  InputPortWidth=4  IndexOptions=Select all,Index vector (dialog)  Indices=4,4  OutputSizes=1,1
  Selector9 : Selector  NumberOfDimensions=2  InputPortWidth=4  IndexOptions=Select all,Index vector (dialog)  Indices=1,1  OutputSizes=1,1
  Terminator{,1..20,22..28} (28 alike) : Terminator
  Fx [1x4] : Outport
  Fy [1x4] : Outport  Port=2
  Fz [1x4] : Outport  Port=3
  Mx [1x4] : Outport  Port=4
  My [1x4] : Outport  Port=5
  Mz [1x4] : Outport  Port=6
  z [1x4] : Outport  Port=7
  zdot [1x4] : Outport  Port=8
  Re [1x4] : Outport  Port=9
  omega [1x4] : Outport  Port=10
  Kappa [1x4] : Outport  Port=11
  Alpha [1x4] : Outport  Port=12
  wires:
  Bus Selector/1 -> Selector/1  "<BrkPrs>"
  Bus Selector/2 -> Selector1/1  "<AxlTrq>"
  Bus Selector/3 -> Selector2/1  "<Vx>"
  Bus Selector/4 -> Selector3/1  "<Vy>"
  Bus Selector/5 -> Selector4/1  "<Camber>"
  Bus Selector/6 -> Selector5/1  "<YawRate>"
  Bus Selector/7 -> Selector6/1  "<Prs>"
  Bus Selector/8 -> Selector7/1  "<Gnd>"
  Bus Selector/9 -> Selector8/1  "<Fext>"
  Bus Selector/10 -> Selector9/1  "<ScaleFctrs>"
  BrkPrs [1x4]/1 -> Bus Creator/1  "BrkPrs"
  AxlTrq [1x4]/1 -> Bus Creator/2  "AxlTrq"
  Vx [1x4]/1 -> Bus Creator/3  "Vx"
  Vy [1x4]/1 -> Bus Creator/4  "Vy"
  Camber [1x4]/1 -> Bus Creator/5  "Camber"
  YawRate [1x4]/1 -> Bus Creator/6  "YawRate"
  Prs [1x4]/1 -> Bus Creator/7  "Prs"
  Gnd [1x4]/1 -> Bus Creator/8  "Gnd"
  Fext [1x4]/1 -> Bus Creator/9  "Fext"
  ScaleFctrs [27x4]/1 -> Bus Creator/10  "ScaleFctrs"
  Bus Creator/1 -> Bus Selector3/1, Bus Selector2/1, Bus Selector1/1, Bus Selector/1
  Bus Selector2/1 -> Selector20/1  "<BrkPrs>"
  Bus Selector2/2 -> Selector21/1  "<AxlTrq>"
  Bus Selector2/3 -> Selector22/1  "<Vx>"
  Bus Selector2/4 -> Selector23/1  "<Vy>"
  Bus Selector2/5 -> Selector24/1  "<Camber>"
  Bus Selector2/6 -> Selector25/1  "<YawRate>"
  Bus Selector2/7 -> Selector26/1  "<Prs>"
  Bus Selector2/8 -> Selector27/1  "<Gnd>"
  Bus Selector2/9 -> Selector28/1  "<Fext>"
  Bus Selector2/10 -> Selector29/1  "<ScaleFctrs>"
  Bus Selector3/1 -> Selector30/1  "<BrkPrs>"
  Bus Selector3/2 -> Selector31/1  "<AxlTrq>"
  Bus Selector3/3 -> Selector32/1  "<Vx>"
  Bus Selector3/4 -> Selector33/1  "<Vy>"
  Bus Selector3/5 -> Selector34/1  "<Camber>"
  Bus Selector3/6 -> Selector35/1  "<YawRate>"
  Bus Selector3/7 -> Selector36/1  "<Prs>"
  Bus Selector3/8 -> Selector37/1  "<Gnd>"
  Bus Selector3/9 -> Selector38/1  "<Fext>"
  Bus Selector3/10 -> Selector39/1  "<ScaleFctrs>"
  Bus Selector1/1 -> Selector10/1  "<BrkPrs>"
  Bus Selector1/2 -> Selector11/1  "<AxlTrq>"
  Bus Selector1/3 -> Selector12/1  "<Vx>"
  Bus Selector1/4 -> Selector13/1  "<Vy>"
  Bus Selector1/5 -> Selector14/1  "<Camber>"
  Bus Selector1/6 -> Selector15/1  "<YawRate>"
  Bus Selector1/7 -> Selector16/1  "<Prs>"
  Bus Selector1/8 -> Selector17/1  "<Gnd>"
  Bus Selector1/9 -> Selector18/1  "<Fext>"
  Bus Selector1/10 -> Selector19/1  "<ScaleFctrs>"
  Combined Slip Wheel 2DOF - FrontLeft/2 -> Terminator/1
  Combined Slip Wheel 2DOF - FrontLeft/4 -> Terminator2/1
  Combined Slip Wheel 2DOF - FrontLeft/5 -> Terminator3/1
  Combined Slip Wheel 2DOF - FrontLeft/6 -> Terminator4/1
  Combined Slip Wheel 2DOF - FrontLeft/7 -> Terminator5/1
  Combined Slip Wheel 2DOF - FrontLeft/8 -> Terminator6/1
  Combined Slip Wheel 2DOF - RearLeft/2 -> Terminator7/1
  Combined Slip Wheel 2DOF - RearLeft/3 -> Terminator8/1
  Combined Slip Wheel 2DOF - RearLeft/4 -> Terminator9/1
  Combined Slip Wheel 2DOF - RearLeft/5 -> Terminator10/1
  Combined Slip Wheel 2DOF - RearLeft/6 -> Terminator11/1
  Combined Slip Wheel 2DOF - RearLeft/7 -> Terminator12/1
  Combined Slip Wheel 2DOF - RearLeft/8 -> Terminator13/1
  Combined Slip Wheel 2DOF - FrontRight/2 -> Terminator14/1
  Combined Slip Wheel 2DOF - FrontRight/3 -> Terminator15/1
  Combined Slip Wheel 2DOF - FrontRight/4 -> Terminator16/1
  Combined Slip Wheel 2DOF - FrontRight/5 -> Terminator17/1
  Combined Slip Wheel 2DOF - FrontRight/6 -> Terminator18/1
  Combined Slip Wheel 2DOF - FrontRight/7 -> Terminator19/1
  Combined Slip Wheel 2DOF - FrontRight/8 -> Terminator20/1
  Combined Slip Wheel 2DOF - RearRight/1 -> Rearrange Signals/4(Info_rr)
  Combined Slip Wheel 2DOF - RearRight/2 -> Terminator22/1
  Combined Slip Wheel 2DOF - RearRight/3 -> Terminator23/1
  Combined Slip Wheel 2DOF - RearRight/4 -> Terminator24/1
  Combined Slip Wheel 2DOF - RearRight/5 -> Terminator25/1
  Combined Slip Wheel 2DOF - RearRight/6 -> Terminator26/1
  Combined Slip Wheel 2DOF - RearRight/7 -> Terminator27/1
  Combined Slip Wheel 2DOF - RearRight/8 -> Terminator28/1
  Combined Slip Wheel 2DOF - FrontLeft/1 -> Bus Selector37/1, Bus Selector29/1, Bus Selector33/1, Rearrange Signals/1(Info_fl)
  Combined Slip Wheel 2DOF - FrontRight/1 -> Rearrange Signals/2(Info_fr)
  Rearrange Signals/8(z) -> z [1x4]/1
  Rearrange Signals/10(Re) -> Re [1x4]/1
  Rearrange Signals/5(Mx) -> Mx [1x4]/1
  Rearrange Signals/4(Fz) -> Fz [1x4]/1
  Rearrange Signals/3(Fy) -> Fy [1x4]/1
  Rearrange Signals/7(Mz) -> Mz [1x4]/1
  Rearrange Signals/6(My) -> My [1x4]/1
  Rearrange Signals/9(zdot) -> zdot [1x4]/1
  Rearrange Signals/2(Fx) -> Fx [1x4]/1
  Rearrange Signals/1(omega) -> omega [1x4]/1
  Combined Slip Wheel 2DOF - FrontLeft/3 -> Terminator1/1
  Bus Selector33/1 -> Scope/1  "<z>"
  Bus Selector37/1 -> Scope/2  "<zdot>"
  Bus Selector29/1 -> Scope/3  "<Re>"
  Bus Selector7/1 -> Scope2/3  "<Re>"
  Bus Selector9/1 -> Scope2/2  "<zdot>"
  Bus Selector8/1 -> Scope2/1  "<z>"
  Combined Slip Wheel 2DOF - RearLeft/1 -> Bus Selector9/1, Bus Selector8/1, Bus Selector7/1, Rearrange Signals/3(Info_rl)
  Rearrange Signals/11(Kappa) -> Kappa [1x4]/1
  Rearrange Signals/12(Alpha) -> Alpha [1x4]/1
  Selector/1 -> Combined Slip Wheel 2DOF - FrontLeft/1
  Selector1/1 -> Combined Slip Wheel 2DOF - FrontLeft/2
  Selector2/1 -> Combined Slip Wheel 2DOF - FrontLeft/3
  Selector3/1 -> Combined Slip Wheel 2DOF - FrontLeft/4
  Selector4/1 -> Combined Slip Wheel 2DOF - FrontLeft/5
  Selector5/1 -> Combined Slip Wheel 2DOF - FrontLeft/6
  Selector6/1 -> Combined Slip Wheel 2DOF - FrontLeft/7
  Selector7/1 -> Combined Slip Wheel 2DOF - FrontLeft/8
  Selector8/1 -> Combined Slip Wheel 2DOF - FrontLeft/9
  Selector9/1 -> Combined Slip Wheel 2DOF - FrontLeft/10
  Selector10/1 -> Combined Slip Wheel 2DOF - RearLeft/1
  Selector11/1 -> Combined Slip Wheel 2DOF - RearLeft/2
  Selector12/1 -> Combined Slip Wheel 2DOF - RearLeft/3
  Selector13/1 -> Combined Slip Wheel 2DOF - RearLeft/4
  Selector14/1 -> Combined Slip Wheel 2DOF - RearLeft/5
  Selector15/1 -> Combined Slip Wheel 2DOF - RearLeft/6
  Selector16/1 -> Combined Slip Wheel 2DOF - RearLeft/7
  Selector17/1 -> Combined Slip Wheel 2DOF - RearLeft/8
  Selector18/1 -> Combined Slip Wheel 2DOF - RearLeft/9
  Selector19/1 -> Combined Slip Wheel 2DOF - RearLeft/10
  Selector20/1 -> Combined Slip Wheel 2DOF - FrontRight/1
  Selector21/1 -> Combined Slip Wheel 2DOF - FrontRight/2
  Selector22/1 -> Combined Slip Wheel 2DOF - FrontRight/3
  Selector23/1 -> Combined Slip Wheel 2DOF - FrontRight/4
  Selector24/1 -> Combined Slip Wheel 2DOF - FrontRight/5
  Selector25/1 -> Combined Slip Wheel 2DOF - FrontRight/6
  Selector26/1 -> Combined Slip Wheel 2DOF - FrontRight/7
  Selector27/1 -> Combined Slip Wheel 2DOF - FrontRight/8
  Selector28/1 -> Combined Slip Wheel 2DOF - FrontRight/9
  Selector29/1 -> Combined Slip Wheel 2DOF - FrontRight/10
  Selector30/1 -> Combined Slip Wheel 2DOF - RearRight/1
  Selector31/1 -> Combined Slip Wheel 2DOF - RearRight/2
  Selector32/1 -> Combined Slip Wheel 2DOF - RearRight/3
  Selector33/1 -> Combined Slip Wheel 2DOF - RearRight/4
  Selector34/1 -> Combined Slip Wheel 2DOF - RearRight/5
  Selector35/1 -> Combined Slip Wheel 2DOF - RearRight/6
  Selector36/1 -> Combined Slip Wheel 2DOF - RearRight/7
  Selector37/1 -> Combined Slip Wheel 2DOF - RearRight/8
  Selector38/1 -> Combined Slip Wheel 2DOF - RearRight/9
  Selector39/1 -> Combined Slip Wheel 2DOF - RearRight/10
